simulink model "YAW_CONTROLLED"  (R2023b)
settings: Solver=VariableStepAuto  StartTime=0.0  StopTime=10.0  RelTol=1e-3
undefined symbols (not defined in the file): D_position, I_omega, P_omega, P_position, tau_set
libraries: slpidlib x2
settings Model: Creator=franc  LastModifiedBy=franc

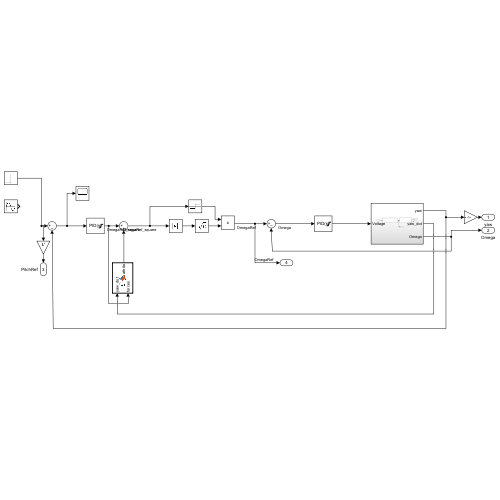
[thumbnail: Simulink's stored preview of the top-level diagram]
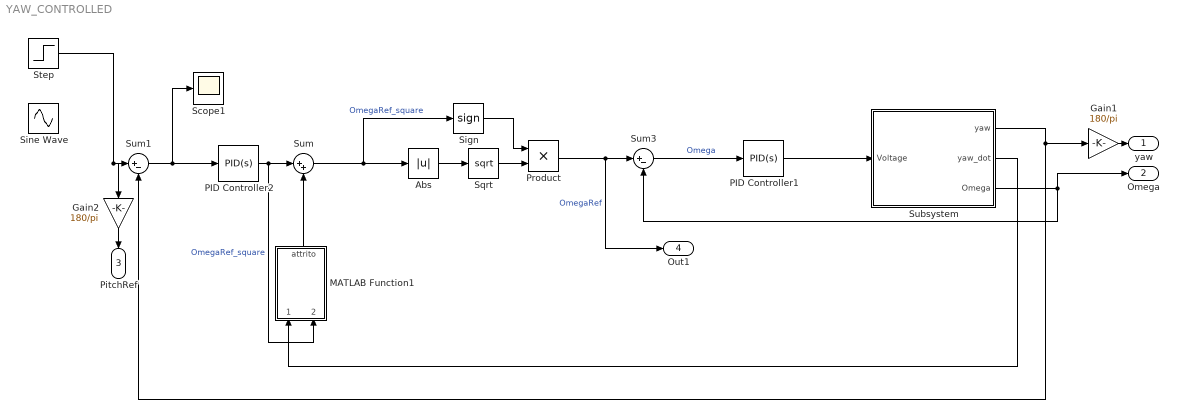
== system YAW_CONTROLLED ==
  Abs : Abs  SaturateOnIntegerOverflow=off
  Gain1 : Gain  Gain=180/pi
  Gain2 : Gain  Gain=180/pi
  MATLAB Function1 : MATLAB Function  TreatAsAtomicUnit=on
  PID Controller1 : slpidlib/PID Controller  Controller=PID  Form=Parallel  TimeDomain=Continuous-time  UseExternalTs=off  SampleTime=-1  IntegratorMethod=Forward Euler  FilterMethod=Forward Euler  ControllerParametersSource=internal  P=P_omega  I=I_omega  UseKiTs=off  D=0  N=100  UseFilter=on  TunerSelectOption=Transfer Function Based (PID Tuner App)  InitialConditionSource=internal  InitialConditionForIntegrator=0  InitialConditionForFilter=0  DifferentiatorICPrevScaledInput=0  ExternalReset=none  TrackingMode=off  Kt=1  LimitOutput=on  SatLimitsSource=internal  UpperSaturationLimit=18  LowerSaturationLimit=-18  LinearizeAsGain=on  AntiWindupMode=none  Kb=1  LimitIntegrator=off  UpperIntegratorSaturationLimit=inf  LowerIntegratorSaturationLimit=-inf  POutMin=[]  POutMax=[]  IOutMin=[]  IOutMax=[]  DOutMin=[]  DOutMax=[]  NOutMin=[]  NOutMax=[]  SumOutMin=[]  SumOutMax=[]  SaturationOutMin=[]  SaturationOutMax=[]  PParamMin=[]  PParamMax=[]  IParamMin=[]  IParamMax=[]  DParamMin=[]  DParamMax=[]  NParamMin=[]  NParamMax=[]  KbParamMin=[]  KbParamMax=[]  KtParamMin=[]  KtParamMax=[]  KbOutMin=[]  KbOutMax=[]  KtOutMin=[]  KtOutMax=[]  IntegratorOutMin=[]  IntegratorOutMax=[]  FilterOutMin=[]  FilterOutMax=[]  SumI1OutMin=[]  SumI1OutMax=[]  SumI2OutMin=[]  SumI2OutMax=[]  SumI3OutMin=[]  SumI3OutMax=[]  SumI4OutMin=[]  SumI4OutMax=[]  SumDOutMin=[]  SumDOutMax=[]  DifferentiatorOutMin=[]  DifferentiatorOutMax=[]  FilterDiffOutCoefMin=[]  FilterDiffOutCoefMax=[]  ReciprocalOutMin=[]  ReciprocalOutMax=[]  SumDenOutMin=[]  SumDenOutMax=[]  SumNumOutMin=[]  SumNumOutMax=[]  DivideOutMin=[]  DivideOutMax=[]  UdiffTsProdOutMin=[]  UdiffTsProdOutMax=[]  NTsProdOutMin=[]  NTsProdOutMax=[]  UintegralTsProdOutMin=[]  UintegralTsProdOutMax=[]  UngainTsProdOutMin=[]  UngainTsProdOutMax=[]  ClampingZeroOutDataTypeStr=Inherit: Inherit via back propagation  ClampingZeroOutMin=[]  ClampingZeroOutMax=[]  FilterDenConstantOutDataTypeStr=Inherit: Inherit via back propagation  FilterDenConstantOutMin=[]  FilterDenConstantOutMax=[]  PCopyOutDataTypeStr=Inherit: Inherit via back propagation  PCopyOutMin=[]  PCopyOutMax=[]  NCopyOutDataTypeStr=Inherit: Inherit via back propagation  NCopyOutMin=[]  NCopyOutMax=[]  IntegratorContinuousStateAttributes=''  IntegratorStateMustResolveToSignalObject=off  IntegratorRTWStateStorageClass=Auto  FilterContinuousStateAttributes=''  FilterStateMustResolveToSignalObject=off  FilterRTWStateStorageClass=Auto  ParallelPVariant=InternalParameters  IdealPVariant=Disabled  IVariant=InternalParameters  DVariant=InternalParameters  IntegratorVariant=Continuous  SatVariant=Enabled  AWVariant=Passthrough  PCopyVariant=Disabled  TRVariant=Disabled  FdbkBlocksVariant=Forward  IdealPFdbkVariant=Disabled  SatFdbkVariant=Disabled  DerivativeFilterVariant=ContFilter  NVariant=InternalParameters  NCopyVariant=Disabled  FilterICVariant=InternalICsFilter  IntegratorICVariant=InternalICs  ExternalResetVariant=Disabled  TRSumVariant=Passthrough  SumFdbkVariant=Disabled  SumVariant=Sum_PID  TsampFilterVariant=InternalTs  TsampNgainVariant=Passthrough  TsampIntegralVariant=Disabled_SignalSpec  ExternalSaturationOutDataTypeStr=Inherit: Same as second input
  PID Controller2 : slpidlib/PID Controller  Controller=PID  Form=Parallel  TimeDomain=Continuous-time  UseExternalTs=off  SampleTime=1/500  IntegratorMethod=Forward Euler  FilterMethod=Forward Euler  ControllerParametersSource=internal  P=P_position*50  I=5000  UseKiTs=off  D=D_position*5  N=1/tau_set  UseFilter=on  TunerSelectOption=Frequency Response Based  InitialConditionSource=internal  InitialConditionForIntegrator=0  InitialConditionForFilter=0  DifferentiatorICPrevScaledInput=0  ExternalReset=none  TrackingMode=off  Kt=1  LimitOutput=on  SatLimitsSource=internal  UpperSaturationLimit=217^2  LowerSaturationLimit=-217^2  LinearizeAsGain=on  AntiWindupMode=clamping  Kb=1  LimitIntegrator=off  UpperIntegratorSaturationLimit=inf  LowerIntegratorSaturationLimit=-inf  POutMin=[]  POutMax=[]  IOutMin=[]  IOutMax=[]  DOutMin=[]  DOutMax=[]  NOutMin=[]  NOutMax=[]  SumOutMin=[]  SumOutMax=[]  SaturationOutMin=[]  SaturationOutMax=[]  PParamMin=[]  PParamMax=[]  IParamMin=[]  IParamMax=[]  DParamMin=[]  DParamMax=[]  NParamMin=[]  NParamMax=[]  KbParamMin=[]  KbParamMax=[]  KtParamMin=[]  KtParamMax=[]  KbOutMin=[]  KbOutMax=[]  KtOutMin=[]  KtOutMax=[]  IntegratorOutMin=[]  IntegratorOutMax=[]  FilterOutMin=[]  FilterOutMax=[]  SumI1OutMin=[]  SumI1OutMax=[]  SumI2OutMin=[]  SumI2OutMax=[]  SumI3OutMin=[]  SumI3OutMax=[]  SumI4OutMin=[]  SumI4OutMax=[]  SumDOutMin=[]  SumDOutMax=[]  DifferentiatorOutMin=[]  DifferentiatorOutMax=[]  FilterDiffOutCoefMin=[]  FilterDiffOutCoefMax=[]  ReciprocalOutMin=[]  ReciprocalOutMax=[]  SumDenOutMin=[]  SumDenOutMax=[]  SumNumOutMin=[]  SumNumOutMax=[]  DivideOutMin=[]  DivideOutMax=[]  UdiffTsProdOutMin=[]  UdiffTsProdOutMax=[]  NTsProdOutMin=[]  NTsProdOutMax=[]  UintegralTsProdOutMin=[]  UintegralTsProdOutMax=[]  UngainTsProdOutMin=[]  UngainTsProdOutMax=[]  ClampingZeroOutDataTypeStr=Inherit: Inherit via back propagation  ClampingZeroOutMin=[]  ClampingZeroOutMax=[]  FilterDenConstantOutDataTypeStr=Inherit: Inherit via back propagation  FilterDenConstantOutMin=[]  FilterDenConstantOutMax=[]  PCopyOutDataTypeStr=Inherit: Inherit via back propagation  PCopyOutMin=[]  PCopyOutMax=[]  NCopyOutDataTypeStr=Inherit: Inherit via back propagation  NCopyOutMin=[]  NCopyOutMax=[]  IntegratorContinuousStateAttributes=''  IntegratorStateMustResolveToSignalObject=off  IntegratorRTWStateStorageClass=Auto  FilterContinuousStateAttributes=''  FilterStateMustResolveToSignalObject=off  FilterRTWStateStorageClass=Auto  ParallelPVariant=InternalParameters  IdealPVariant=Disabled  IVariant=InternalParameters  DVariant=InternalParameters  IntegratorVariant=Continuous  SatVariant=Enabled  AWVariant=ContClampingParallel  PCopyVariant=Disabled  TRVariant=Disabled  FdbkBlocksVariant=Forward  IdealPFdbkVariant=Disabled  SatFdbkVariant=Disabled  DerivativeFilterVariant=ContFilter  NVariant=InternalParameters  NCopyVariant=Disabled  FilterICVariant=InternalICsFilter  IntegratorICVariant=InternalICs  ExternalResetVariant=Disabled  TRSumVariant=Passthrough  SumFdbkVariant=Disabled  SumVariant=Sum_PID  TsampFilterVariant=InternalTs  TsampNgainVariant=Passthrough  TsampIntegralVariant=Disabled_SignalSpec  ExternalSaturationOutDataTypeStr=Inherit: Same as second input
  Product : Product
  Scope1 : Scope
  Sign : Signum
  Sine Wave : Sin  Frequency=2*pi/12  SampleTime=0
  Sqrt : Sqrt
  Step : Step  After=30*pi/180  SampleTime=0
  Subsystem : Subsystem
  Sum : Sum  Inputs=|++
  Sum1 : Sum  Inputs=|+-
  Sum3 : Sum  Inputs=|+-
  yaw : Outport
  Omega : Outport  Port=2
  PitchRef : Outport  Port=3
  Out1 : Outport  Port=4
  wires:
  Sum1/1 -> PID Controller2/1, Scope1/1
  Step/1 -> Gain2/1, Sum1/1
  Abs/1 -> Sqrt/1
  Product/1 -> Sum3/1, Out1/1  "OmegaRef"
  Subsystem/1(yaw) -> Sum1/2, Gain1/1
  Sqrt/1 -> Product/2
  Sum3/1 -> PID Controller1/1  "Omega"
  Subsystem/3(Omega) -> Omega/1, Sum3/2
  Gain1/1 -> yaw/1
  Gain2/1 -> PitchRef/1
  Sum/1 -> Abs/1, Sign/1  "OmegaRef_square"
  Sign/1 -> Product/1
  PID Controller1/1 -> Subsystem/1(Voltage)
  PID Controller2/1 -> Sum/1, MATLAB Function1/2(forces)  "OmegaRef_square"
  Subsystem/2(yaw_dot) -> MATLAB Function1/1(yaw_dot)
  MATLAB Function1/1(attrito) -> Sum/2

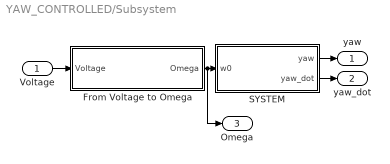
== system YAW_CONTROLLED/Subsystem ==
  Voltage : Inport
  From Voltage to Omega : Subsystem
  SYSTEM : Subsystem
  yaw : Outport
  yaw_dot : Outport  Port=2
  Omega : Outport  Port=3
  wires:
  From Voltage to Omega/1(Omega) -> Omega/1, SYSTEM/1(w0)
  SYSTEM/1(yaw) -> yaw/1
  SYSTEM/2(yaw_dot) -> yaw_dot/1
  Voltage/1 -> From Voltage to Omega/1(Voltage)

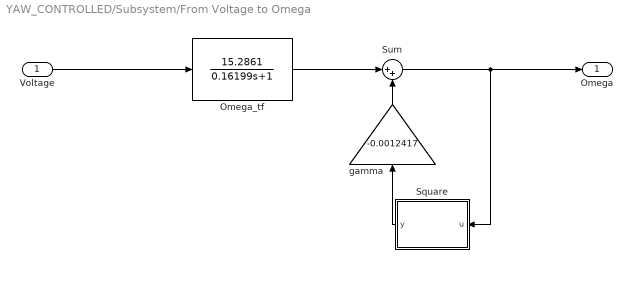
== system YAW_CONTROLLED/Subsystem/From Voltage to Omega ==
  Voltage : Inport
  Omega_tf : TransferFcn  Numerator=15.2861  Denominator=[0.16199 1]
  Square : MATLAB Function  TreatAsAtomicUnit=on
  Sum : Sum  Inputs=|++
  gamma : Gain  Gain=-0.0012417
  Omega : Outport
  wires:
  Voltage/1 -> Omega_tf/1
  gamma/1 -> Sum/2
  Square/1(y) -> gamma/1
  Omega_tf/1 -> Sum/1
  Sum/1 -> Omega/1, Square/1(u)

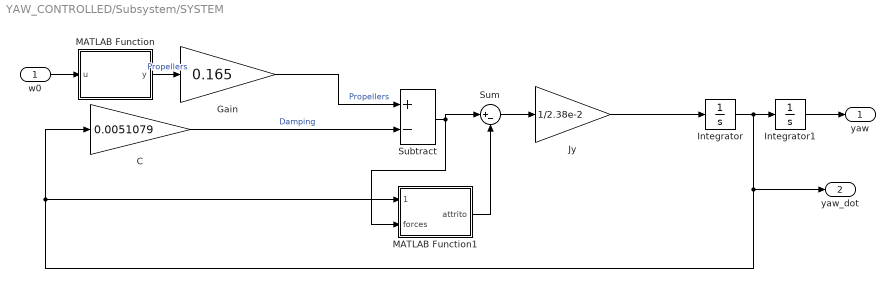
== system YAW_CONTROLLED/Subsystem/SYSTEM ==
  w0 : Inport
  C : Gain  Gain=0.0051079
  Gain : Gain  Gain=0.165
  Integrator : Integrator
  Integrator1 : Integrator
  Jy : Gain  Gain=1/2.38e-2
  MATLAB Function : MATLAB Function  TreatAsAtomicUnit=on
  MATLAB Function1 : MATLAB Function  TreatAsAtomicUnit=on
  Subtract : Sum  Inputs=+-
  Sum : Sum  Inputs=|+-
  yaw : Outport
  yaw_dot : Outport  Port=2
  wires:
  Jy/1 -> Integrator/1
  Gain/1 -> Subtract/1  "Propellers"
  Integrator1/1 -> yaw/1
  Integrator/1 -> Integrator1/1, yaw_dot/1, MATLAB Function1/1(yaw_dot), C/1
  Subtract/1 -> Sum/1, MATLAB Function1/2(forces)
  C/1 -> Subtract/2  "Damping"
  w0/1 -> MATLAB Function/1(u)
  MATLAB Function/1(y) -> Gain/1  "Propellers"
  Sum/1 -> Jy/1
  MATLAB Function1/1(attrito) -> Sum/2

== matlab function YAW_CONTROLLED/Subsystem/SYSTEM/MATLAB Function ==
  data: u input; y output
function y = fcn(u)
y = -2.522922e-05*u+4.01487e-06*u^2*sign(u);

== matlab function YAW_CONTROLLED/Subsystem/From Voltage to Omega/Square ==
  data: u input; y output
function y = fcn(u)
y=u^2*sign(u);

== matlab function YAW_CONTROLLED/MATLAB Function1 ==
  data: yaw_dot input; attrito output; forces input
function attrito = fcn(yaw_dot,forces)
fd=0.0035;
fs=0.0088;

attrito=abs(forces);

if attrito>fs || abs(yaw_dot)>=1
    attrito=fd;
end

attrito=attrito*sign(yaw_dot);

== matlab function YAW_CONTROLLED/Subsystem/SYSTEM/MATLAB Function1 ==
  data: yaw_dot input; attrito output; forces input
function attrito = fcn(yaw_dot,forces)
fd=0.0035;
fs=0.0088;

attrito=abs(forces);

if attrito>fs || abs(yaw_dot)>=1
    attrito=fd;
end
attrito=attrito*sign(yaw_dot);
